simulink model "LeftArmAgent"  (Simulink 7.1)
settings: Solver=ode45  SolverMode=SingleTasking  StartTime=0.0  StopTime=10.0  RelTol=1e-3  AbsTol=1e-6
settings Model: Creator=The MathWorks Inc.  LastModifiedBy=luox2  ExtModeTrigMode=oneshot  ExtModeArmWhenConnect=off  ExtModeAutoUpdateStatusClock=off
settings DataIOCC: LimitDataPoints=off  SignalLoggingName=logsOut
settings OptimizationCC: BooleanDataType=off  InlineInvariantSignals=on
settings DebuggingCC: SaveWithParameterizedLinksMsg=none  CheckExecutionContextPreStartOutputMsg=on  CheckExecutionContextRuntimeOutputMsg=on  SignalResolutionControl=TryResolveAllWithWarning  SolverPrmCheckMsg=none  MultiTaskDSMMsg=warning  MultiTaskCondExecSysMsg=none  IntegerOverflowMsg=none  StrictBusMsg=None
settings HardwareCC: TargetUnknown=on
settings ModelReferenceCC: UpdateModelReferenceTargets=IfOutOfDate
settings RTWCC: IncludeERTFirstTime=on
settings GRTTargetCC: TargetFcnLib=ansi_tfl_tmw.mat

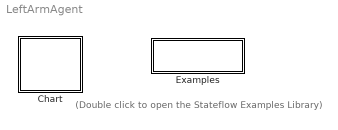
== system LeftArmAgent ==
  note: (Double click to open the
      | Stateflow Examples Library)
  Chart : Stateflow chart
  Examples : Subsystem
      settings: OpenFcn=sf('Private','sf_examples')
      mask Display: disp('Examples')

== system LeftArmAgent/Examples ==

== stateflow chart Chart ==
  state InitialArmRoutine
    HungerForce\LeftReachDemo\LeftArm\HomingController.ComputeHomingPressures()
    HungerForce\LeftReachDemo\LeftArm\SampleIndPressure.HW_IO_6()
    HungerForce\LeftReachDemo\LeftArm\StateMachine.Wait(50)
  state InitializeFunctions
    HungerForce\LeftReachDemo\LeftArm\HomingController.Initial()
    HungerForce\LeftReachDemo\LeftArm\SampleIndPressure.Initialize()
    HungerForce\LeftReachDemo\LeftArm\PIDNonLinCtrl.Initial()
    HungerForce\LeftReachDemo\LeftArm\ForwardKinematics.Initialize()
    HungerForce\LeftReachDemo\LeftArm\InverseKinematics.Initialize()
    HungerForce\LeftReachDemo\LeftArm\SampleIndPressure.Disable_ZMasking()
  state WriteHomeDesiredLogicalAngles
    HungerForce\LeftReachDemo\LeftArm\SampleIndPressure.Enable_ZMasking()
    HungerForce\LeftReachDemo\LeftArm\SampleIndPressure.WriteHomePositions()
  state LoadHomePosition
    HungerForce\LeftReachDemo\LeftArm\SampleIndPressure.HW_IO_6()
    HungerForce\LeftReachDemo\LeftArm\PIDNonLinCtrl.PID_NonLin_6Press()
    HungerForce\LeftReachDemo\LeftArm\ForwardKinematics.ForwardKinematics()
    HungerForce\LeftReachDemo\LeftArm\InverseKinematics.InverseKinematics()
  state PID_NonLinCtrlLoop
    HungerForce\LeftReachDemo\LeftArm\Filter.FilterDesiredAngles()
    HungerForce\LeftReachDemo\LeftArm\PIDNonLinCtrl.PID_NonLin_12Press()
    HungerForce\LeftReachDemo\LeftArm\SampleIndPressure.HW_IO_12()
    HungerForce\LeftReachDemo\LeftArm\PIDNonLinCtrl.Read_CurrentPressure()
    HungerForce\LeftReachDemo\LeftArm\ForwardKinematics.ForwardKinematics()
    HungerForce\LeftReachDemo\LeftArm\InverseKinematics.InverseKinematics()
    HungerForce\LeftReachDemo\LeftArm\StateMachine.Wait(50)
  state Fire event to start Trajectory Generation in Popeye
    HungerForce\LeftReachDemo\LeftTrajectoryAgent\StateMachine.LoadSM()
    HungerForce\LeftReachDemo\LeftTrajectoryAgent\StateMachine.Start()
  (default) -> InitializeFunctions : Start
  InitialArmRoutine -> InitialArmRoutine [order 1] : Default
  InitializeFunctions -> InitialArmRoutine : Always
  WriteHomeDesiredLogicalAngles -> LoadHomePosition : Always
  LoadHomePosition -> Fire event to start Trajectory Generation in Popeye : Always
  InitialArmRoutine -> WriteHomeDesiredLogicalAngles [order 2] : Signal="Go to next state"
  PID_NonLinCtrlLoop -> PID_NonLinCtrlLoop : Default
  Fire event to start Trajectory Generation in Popeye -> PID_NonLinCtrlLoop : Always
